simulink model "PMSM_FOC_VOPEN"  (R2022a)
settings: Solver=FixedStepAuto  StartTime=0.0  StopTime=0.5  FixedStep=Ts  RelTol=1e-3
undefined symbols (not defined in the file): pmsm, Ts
libraries: mcbcontrolslib x3, mcbplantlib x1, autolibpmsmexterior x1, eeGeneralControl x1
settings Model: Creator=徐国强  LastModifiedBy=徐国强

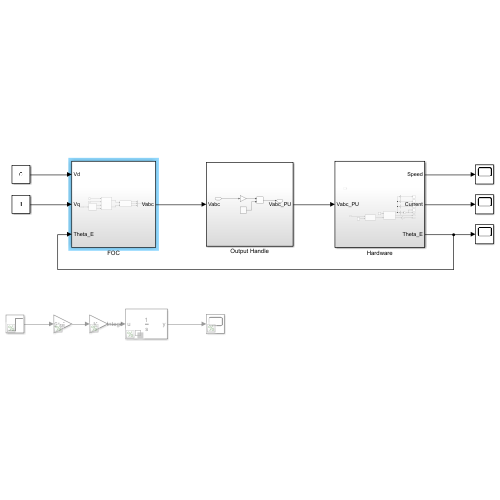
[thumbnail: Simulink's stored preview of the top-level diagram]
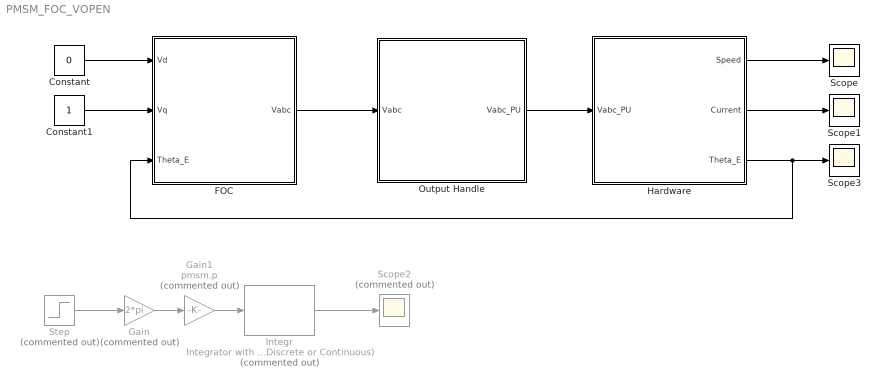
== system PMSM_FOC_VOPEN ==
  Constant : Constant  Value=0
  Constant1 : Constant
  FOC : Subsystem
  Gain : Gain  Commented=on  Gain=2*pi
  Gain1 : Gain  Commented=on  Gain=pmsm.p
  Hardware : Subsystem
  Integr : eeGeneralControl/Integrator with Wrapped State (Discrete or Continuous)  Commented=on  LabelModeActiveChoice=Discrete  WrappedStateUpperValue=pi*pmsm.p  WrappedStateLowerValue=-pi*pmsm.p  x0=0  Ts=Ts
      settings: SourceProductBaseCode=PS
  Output Handle : Subsystem
  Scope : Scope
  Scope1 : Scope
  Scope2 : Scope  Commented=on
  Scope3 : Scope
  Step : Step  Commented=on  Time=0  After=51.468  SampleTime=0
  wires:
  Hardware/2(Current) -> Scope1/1
  Constant/1 -> FOC/1(Vd)
  Hardware/1(Speed) -> Scope/1
  FOC/1(Vabc) -> Output Handle/1(Vabc)
  Output Handle/1(Vabc_PU) -> Hardware/1(Vabc_PU)
  Constant1/1 -> FOC/2(Vq)
  Step/1 -> Gain/1
  Hardware/3(Theta_E) -> FOC/3(Theta_E), Scope3/1
  Integr/1 -> Scope2/1
  Gain/1 -> Gain1/1
  Gain1/1 -> Integr/1

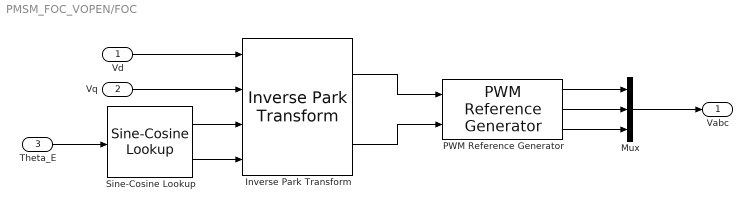
== system PMSM_FOC_VOPEN/FOC ==
  Vd : Inport
  Vq : Inport  Port=2
  Theta_E : Inport  Port=3
  Inverse Park Transform : mcbcontrolslib/Inverse Park Transform  AxisAlignment=D-axis
  Mux : Mux  Inputs=3
  PWM Reference Generator : mcbcontrolslib/PWM Reference Generator  inSignal=Valphabeta  modType=SVM: space vector modulation
      settings: SourceProductBaseCode=MT
  Sine-Cosine Lookup : mcbcontrolslib/Sine-Cosine Lookup  AngleInput=Radians  N_points=1024
      settings: SourceProductBaseCode=MT
  Vabc : Outport
  wires:
  Theta_E/1 -> Sine-Cosine Lookup/1
  Vd/1 -> Inverse Park Transform/1
  Mux/1 -> Vabc/1
  PWM Reference Generator/3 -> Mux/3
  Sine-Cosine Lookup/2 -> Inverse Park Transform/4
  PWM Reference Generator/2 -> Mux/2
  PWM Reference Generator/1 -> Mux/1
  Sine-Cosine Lookup/1 -> Inverse Park Transform/3
  Inverse Park Transform/2 -> PWM Reference Generator/2
  Inverse Park Transform/1 -> PWM Reference Generator/1
  Vq/1 -> Inverse Park Transform/2

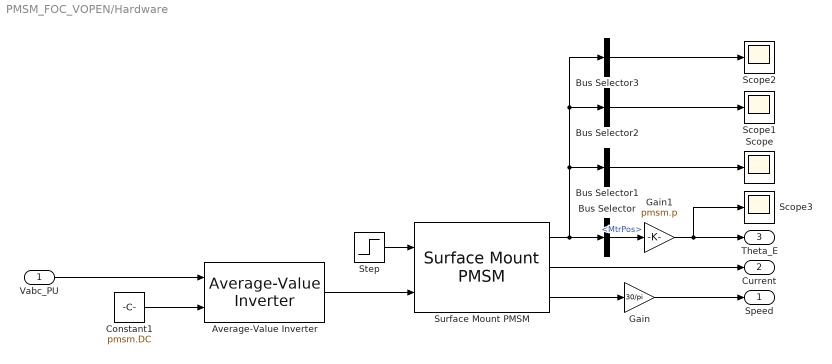
== system PMSM_FOC_VOPEN/Hardware ==
  Vabc_PU : Inport
  Average-Value Inverter : mcbplantlib/Average-Value Inverter
  Bus Selector : BusSelector  OutputSignals=MtrPos
  Bus Selector1 : BusSelector  OutputSignals=IdSync,IqSync  OutputAsBus=on
  Bus Selector2 : BusSelector  OutputSignals=VdSync,VqSync  OutputAsBus=on
  Bus Selector3 : BusSelector  OutputSignals=MtrTrq  OutputAsBus=on
  Constant1 : Constant  Value=pmsm.DC
  Gain : Gain  Gain=30/pi
  Gain1 : Gain  Gain=pmsm.p
  Scope{,1..3} (4 alike) : Scope
  Step : Step  Time=0.2  After=0.05*pmsm.T_rated  SampleTime=0
  Surface Mount PMSM : autolibpmsmexterior/Surface Mount PMSM  port_config=Torque  sim_type=Discrete  Ts=Ts  P=pmsm.p  Rs=pmsm.Rs  Ldq_=pmsm.Ld  KConstText=Permanent flux linkage constant (lambda_pm):  lambda_pm=pmsm.FluxPM  Ke=159.9771  Kt=1.323  mechanical=[pmsm.J, pmsm.B, 0]  idq0=[0 0]  theta_init=0  omega_init=0  KConst=pmsm.FluxPM  lambda_pm_calc=pmsm.FluxPM  RefBlkName='autolibpmsmexterior/Surface Mount PMSM'  aMode=5  Ldq="[0.0017      0.0017]"
      settings: SourceProductBaseCode=PW,DR,MT,VE
  Speed : Outport
  Current : Outport  Port=2
  Theta_E : Outport  Port=3
  wires:
  Vabc_PU/1 -> Average-Value Inverter/1
  Gain1/1 -> Scope3/1, Theta_E/1
  Surface Mount PMSM/1 -> Bus Selector3/1, Bus Selector2/1, Bus Selector1/1, Bus Selector/1
  Surface Mount PMSM/3 -> Gain/1
  Average-Value Inverter/1 -> Surface Mount PMSM/2
  Surface Mount PMSM/2 -> Current/1
  Gain/1 -> Speed/1
  Constant1/1 -> Average-Value Inverter/2
  Bus Selector/1 -> Gain1/1  "<MtrPos>"
  Bus Selector1/1 -> Scope/1
  Bus Selector2/1 -> Scope1/1
  Bus Selector3/1 -> Scope2/1
  Step/1 -> Surface Mount PMSM/1

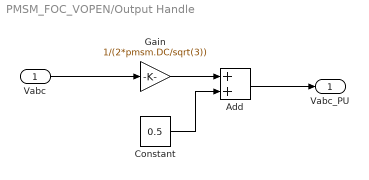
== system PMSM_FOC_VOPEN/Output Handle ==
  Vabc : Inport
  Add : Sum
  Constant : Constant  Value=0.5
  Gain : Gain  Gain=1/(2*pmsm.DC/sqrt(3))
  Vabc_PU : Outport
  wires:
  Constant/1 -> Add/2
  Add/1 -> Vabc_PU/1
  Gain/1 -> Add/1
  Vabc/1 -> Gain/1
